simulink model "Crazyflie_TrajectoryTracking"  (R2020b)
settings: Solver=ode15s  StartTime=0.0  StopTime=100  MaxStep=1.0  RelTol=1e-5
settings Model: Creator=iketa  LastModifiedBy=kt012
settings DataIOCC: ReturnWorkspaceOutputs=off
settings DebuggingCC: ArithmeticOperatorsInVariantConditions=warning
settings SFSimCC: CustomCodeUndefinedFunction=UseInterfaceOnly

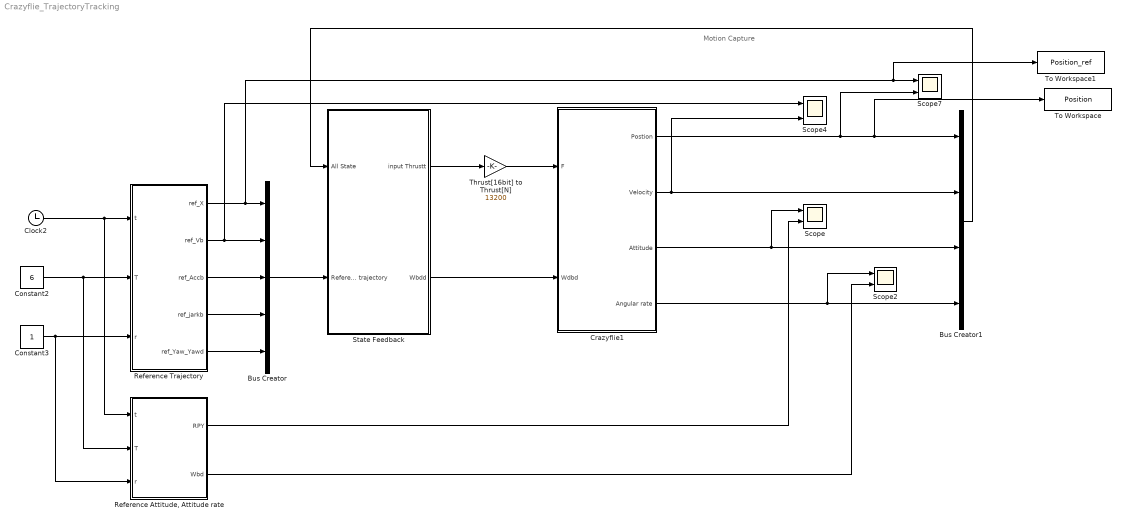
== system Crazyflie_TrajectoryTracking ==
  note: Motion Capture
  Bus Creator : BusCreator  Inputs=5
  Bus Creator1 : BusCreator  Inputs=Position,Body velosity,Euler_angle,Body anglar velosity
  Clock2 : Clock
  Constant2 : Constant  Value=6
  Constant3 : Constant
  Crazyflie1 : Subsystem
  "Reference Attitude, Attitude rate " : MATLAB Function  TreatAsAtomicUnit=on
  Reference Trajectory : MATLAB Function  TreatAsAtomicUnit=on
  Scope{,2,4,7} (4 alike) : Scope  NumInputPorts=2
  State Feedback : Subsystem
  Thrust[16bit] to Thrust[N] : Gain  Gain=13200
  To Workspace : ToWorkspace  VariableName=Position  SaveFormat=Timeseries  SampleTime=-1
  To Workspace1 : ToWorkspace  VariableName=Position_ref  SaveFormat=Timeseries  SampleTime=-1
  wires:
  Crazyflie1/2(Velocity) -> Bus Creator1/2, Scope4/2
  State Feedback/2("Wbdd ") -> Crazyflie1/2(Wdbd)
  Crazyflie1/3(Attitude) -> Scope/1, Bus Creator1/3
  Crazyflie1/4(Angular rate) -> Bus Creator1/4, Scope2/1
  Crazyflie1/1(Postion) -> Scope7/2, Bus Creator1/1, To Workspace/1
  Constant2/1 -> Reference Trajectory/2(T), "Reference Attitude, Attitude rate "/2(T)
  Constant3/1 -> Reference Trajectory/3(r), "Reference Attitude, Attitude rate "/3(r)
  Clock2/1 -> Reference Trajectory/1(t), "Reference Attitude, Attitude rate "/1(t)
  Reference Trajectory/3(ref_Accb) -> Bus Creator/3
  Bus Creator1/1 -> State Feedback/1(All State)
  Reference Trajectory/2(ref_Vb) -> Scope4/1, Bus Creator/2
  Reference Trajectory/1(ref_X) -> To Workspace1/1, Scope7/1, Bus Creator/1
  Thrust[16bit] to Thrust[N]/1 -> Crazyflie1/1(F)
  Reference Trajectory/5(ref_Yaw_Yawd) -> Bus Creator/5
  Bus Creator/1 -> State Feedback/2(Reference trajectory)
  State Feedback/1(input Thrustt) -> Thrust[16bit] to Thrust[N]/1
  Reference Trajectory/4(ref_jarkb) -> Bus Creator/4
  "Reference Attitude, Attitude rate "/2(Wbd) -> Scope2/2
  "Reference Attitude, Attitude rate "/1(RPY) -> Scope/2

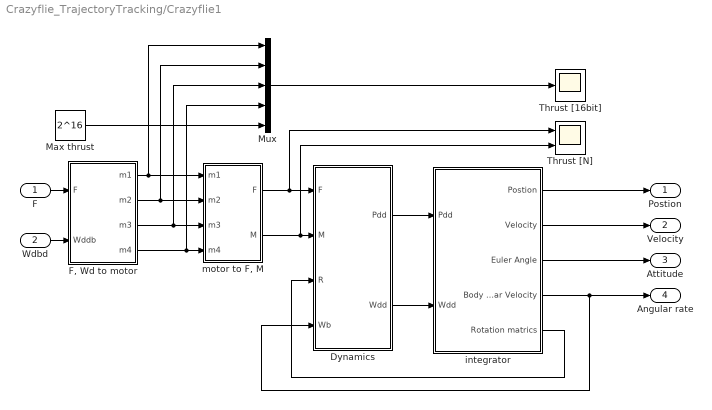
== system Crazyflie_TrajectoryTracking/Crazyflie1 ==
  F : Inport
  Wdbd : Inport  Port=2
  Dynamics : MATLAB Function  TreatAsAtomicUnit=on
  "F, Wd to motor" : MATLAB Function  TreatAsAtomicUnit=on
  Max thrust : Constant  Value=2^16
  Mux : Mux  Inputs=5
  "Thrust [16bit] " : Scope
  Thrust [N] : Scope  NumInputPorts=2
  integrator : Subsystem
  "motor to F, M" : MATLAB Function  TreatAsAtomicUnit=on
  Postion : Outport
  Velocity : Outport  Port=2
  Attitude : Outport  Port=3
  Angular rate : Outport  Port=4
  wires:
  "F, Wd to motor"/1(m1) -> "motor to F, M"/1(m1), Mux/1
  Wdbd/1 -> "F, Wd to motor"/2(Wddb)
  "F, Wd to motor"/4(m4) -> Mux/4, "motor to F, M"/4(m4)
  "F, Wd to motor"/2(m2) -> "motor to F, M"/2(m2), Mux/2
  "F, Wd to motor"/3(m3) -> "motor to F, M"/3(m3), Mux/3
  Dynamics/2(Wdd) -> integrator/2(Wdd)
  "motor to F, M"/2(M) -> Thrust [N]/2, Dynamics/2(M)
  integrator/4(Body Angular Velocity) -> Dynamics/4(Wb), Angular rate/1
  "motor to F, M"/1(F) -> Thrust [N]/1, Dynamics/1(F)
  F/1 -> "F, Wd to motor"/1(F)
  Dynamics/1(Pdd) -> integrator/1(Pdd)
  integrator/1(Postion) -> Postion/1
  integrator/2(Velocity) -> Velocity/1
  Mux/1 -> "Thrust [16bit] "/1
  Max thrust/1 -> Mux/5
  integrator/5(Rotation matrics) -> Dynamics/3(R)
  integrator/3(Euler Angle) -> Attitude/1

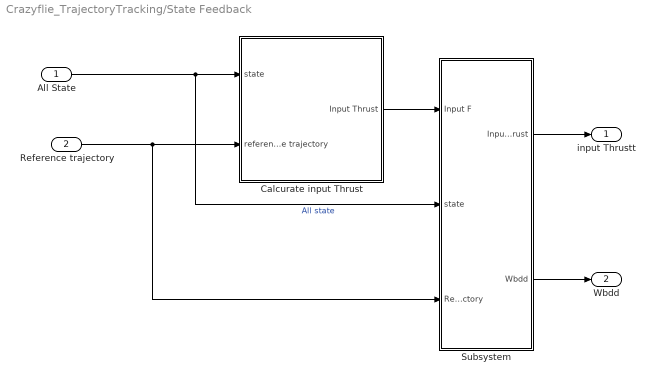
== system Crazyflie_TrajectoryTracking/State Feedback ==
  All State : Inport
  Reference trajectory : Inport  Port=2
  Calcurate input Thrust : Subsystem
  Subsystem : Subsystem
  input Thrustt : Outport
  "Wbdd " : Outport  Port=2  VectorParamsAs1DForOutWhenUnconnected=off
  wires:
  All State/1 -> Subsystem/2(state), Calcurate input Thrust/1(state)  "All state"
  Reference trajectory/1 -> Subsystem/3(Reference Trajectory), Calcurate input Thrust/2(reference trajectory)
  Calcurate input Thrust/1(Input Thrust) -> Subsystem/1(Input F)
  Subsystem/2("Wbdd ") -> "Wbdd "/1
  Subsystem/1(Input Thrust) -> input Thrustt/1

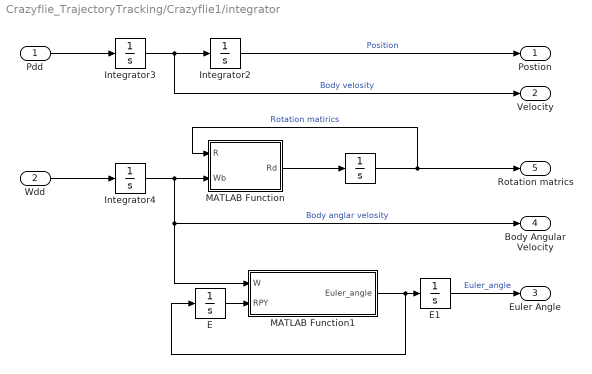
== system Crazyflie_TrajectoryTracking/Crazyflie1/integrator ==
  Pdd : Inport
  Wdd : Inport  Port=2
  " " : Integrator  InitialCondition=[1 0 0; 0 1 0; 0 0 1];  ContinuousStateAttributes="\"\""
  E : Integrator  InitialCondition=[0 0 0];
  E1 : Integrator  InitialCondition=[0 0 0];
  Integrator2 : Integrator  InitialCondition=[0 0.5 0];
  Integrator3 : Integrator  InitialCondition=[0 0 0.0];
  Integrator4 : Integrator  InitialCondition=[0 0 0];  ContinuousStateAttributes='Body_anglar_velocity'
  MATLAB Function : MATLAB Function  TreatAsAtomicUnit=on
  MATLAB Function1 : MATLAB Function  TreatAsAtomicUnit=on
  Postion : Outport
  Velocity : Outport  Port=2
  Euler Angle : Outport  Port=3
  Body Angular Velocity : Outport  Port=4
  Rotation matrics : Outport  Port=5
  wires:
  Integrator4/1 -> Body Angular Velocity/1, MATLAB Function1/1(W), MATLAB Function/2(Wb)  "Body anglar velosity"
  Pdd/1 -> Integrator3/1
  Integrator3/1 -> Integrator2/1, Velocity/1  "Body velosity"
  Integrator2/1 -> Postion/1  "Position"
  Wdd/1 -> Integrator4/1
  " "/1 -> MATLAB Function/1(R), Rotation matrics/1  "Rotation matirics"
  MATLAB Function/1(Rd) -> " "/1
  E/1 -> MATLAB Function1/2(RPY)
  MATLAB Function1/1(Euler_angle) -> E/1, E1/1
  E1/1 -> Euler Angle/1  "Euler_angle"

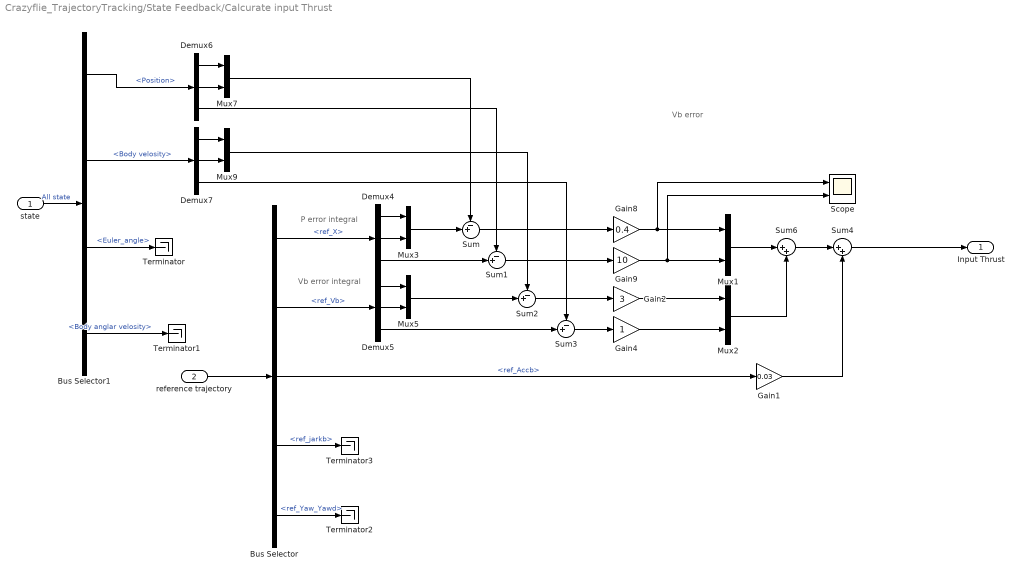
== system Crazyflie_TrajectoryTracking/State Feedback/Calcurate input Thrust ==
  note: Vb error
  note: P error integral
  note: Vb error integral
  state : Inport
  reference trajectory : Inport  Port=2
  Bus Selector : BusSelector  OutputSignals=ref_X,ref_Vb,ref_Accb,ref_jarkb,ref_Yaw_Yawd
  Bus Selector1 : BusSelector  OutputSignals=Position,Body velosity,Euler_angle,Body anglar velosity
  Demux{4..7} (4 alike) : Demux  Outputs=3
  Gain1 : Gain  Gain=0.03
  Gain2 : Gain  Gain=3
  Gain4 : Gain
  Gain8 : Gain  Gain=0.4
  Gain9 : Gain  Gain=10
  Mux{1..3,5,7,9} (6 alike) : Mux  Inputs=2
  Scope : Scope  NumInputPorts=2
  Sum{,1..3} (4 alike) : Sum  Inputs=-+|
  Sum4 : Sum  Inputs=|++
  Sum6 : Sum  Inputs=|++
  Terminator{,1..3} (4 alike) : Terminator
  Input Thrust : Outport
  wires:
  Gain9/1 -> Scope/2, Mux1/2
  Demux5/1 -> Mux5/1
  Gain8/1 -> Scope/1, Mux1/1
  Demux7/3 -> Sum3/1
  Bus Selector/2 -> Demux5/1  "<ref_Vb>"
  Demux5/2 -> Mux5/2
  Mux7/1 -> Sum/1
  Mux9/1 -> Sum2/1
  Sum2/1 -> Gain2/1
  Sum6/1 -> Sum4/1
  Demux7/2 -> Mux9/2
  Demux4/2 -> Mux3/2
  Sum1/1 -> Gain9/1
  Demux6/2 -> Mux7/2
  Demux6/3 -> Sum1/1
  Gain4/1 -> Mux2/2
  Sum/1 -> Gain8/1
  Demux4/1 -> Mux3/1
  Mux2/1 -> Sum6/2
  Demux4/3 -> Sum1/2
  reference trajectory/1 -> Bus Selector/1
  Sum3/1 -> Gain4/1
  Gain2/1 -> Mux2/1
  Mux1/1 -> Sum6/1
  Demux6/1 -> Mux7/1
  Gain1/1 -> Sum4/2
  state/1 -> Bus Selector1/1  "All state"
  Bus Selector1/4 -> Terminator1/1  "<Body anglar velosity>"
  Bus Selector1/2 -> Demux7/1  "<Body velosity>"
  Mux5/1 -> Sum2/2
  Mux3/1 -> Sum/2
  Demux5/3 -> Sum3/2
  Bus Selector1/3 -> Terminator/1  "<Euler_angle>"
  Demux7/1 -> Mux9/1
  Bus Selector1/1 -> Demux6/1  "<Position>"
  Sum4/1 -> Input Thrust/1
  Bus Selector/3 -> Gain1/1  "<ref_Accb>"
  Bus Selector/1 -> Demux4/1  "<ref_X>"
  Bus Selector/5 -> Terminator2/1  "<ref_Yaw_Yawd>"
  Bus Selector/4 -> Terminator3/1  "<ref_jarkb>"

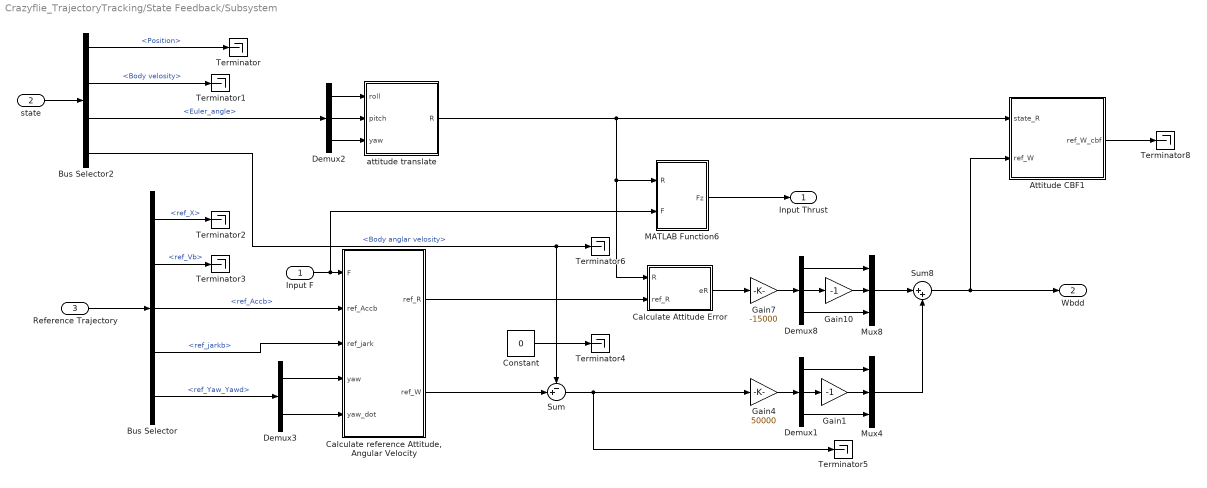
== system Crazyflie_TrajectoryTracking/State Feedback/Subsystem ==
  Input F : Inport
  state : Inport  Port=2
  Reference Trajectory : Inport  Port=3
  Attitude CBF1 : MATLAB Function  TreatAsAtomicUnit=on
  Bus Selector : BusSelector  OutputSignals=ref_X,ref_Vb,ref_Accb,ref_jarkb,ref_Yaw_Yawd
  Bus Selector2 : BusSelector  OutputSignals=Position,Body velosity,Euler_angle,Body anglar velosity
  Calculate Attitude Error : MATLAB Function  TreatAsAtomicUnit=on
  "Calculate reference Attitude, Angular Velocity" : MATLAB Function  TreatAsAtomicUnit=on
  Constant : Constant  Value=0
  Demux1 : Demux  Outputs=3
  Demux2 : Demux  Outputs=3
  Demux3 : Demux  Outputs=2
  Demux8 : Demux  Outputs=3
  Gain1 : Gain  Gain=-1
  Gain10 : Gain  Gain=-1
  Gain4 : Gain  Gain=50000
  Gain7 : Gain  Gain=-15000
  MATLAB Function6 : MATLAB Function
  Mux4 : Mux  Inputs=3
  Mux8 : Mux  Inputs=3
  Sum : Sum  Inputs=-+|
  Sum8 : Sum  Inputs=|++
  Terminator{,1..6,8} (8 alike) : Terminator
  attitude translate : MATLAB Function  TreatAsAtomicUnit=on
  Input Thrust : Outport
  "Wbdd " : Outport  Port=2  VectorParamsAs1DForOutWhenUnconnected=off
  wires:
  Sum/1 -> Gain4/1, Terminator5/1
  Mux4/1 -> Sum8/2
  Bus Selector/2 -> Terminator3/1  "<ref_Vb>"
  Demux8/3 -> Mux8/3
  "Calculate reference Attitude, Angular Velocity"/1(ref_R) -> Calculate Attitude Error/2(ref_R)
  Mux8/1 -> Sum8/1
  Sum8/1 -> "Wbdd "/1, Attitude CBF1/2(ref_W)
  Input F/1 -> MATLAB Function6/2(F), "Calculate reference Attitude, Angular Velocity"/1(F)
  Demux8/2 -> Gain10/1
  attitude translate/1(R) -> Attitude CBF1/1(state_R), Calculate Attitude Error/1(R), MATLAB Function6/1(R)
  Demux8/1 -> Mux8/1
  Gain10/1 -> Mux8/2
  Demux1/2 -> Gain1/1
  Bus Selector2/3 -> Demux2/1  "<Euler_angle>"
  Bus Selector2/2 -> Terminator1/1  "<Body velosity>"
  Bus Selector2/1 -> Terminator/1  "<Position>"
  Bus Selector/5 -> Demux3/1  "<ref_Yaw_Yawd>"
  Bus Selector2/4 -> Terminator6/1, Sum/1  "<Body anglar velosity>"
  Reference Trajectory/1 -> Bus Selector/1
  Bus Selector/3 -> "Calculate reference Attitude, Angular Velocity"/2(ref_Accb)  "<ref_Accb>"
  "Calculate reference Attitude, Angular Velocity"/2(ref_W) -> Sum/2
  Demux3/1 -> "Calculate reference Attitude, Angular Velocity"/4(yaw)
  Calculate Attitude Error/1(eR) -> Gain7/1
  Demux3/2 -> "Calculate reference Attitude, Angular Velocity"/5(yaw_dot)
  state/1 -> Bus Selector2/1
  MATLAB Function6/1(Fz) -> Input Thrust/1
  Bus Selector/1 -> Terminator2/1  "<ref_X>"
  Bus Selector/4 -> "Calculate reference Attitude, Angular Velocity"/3(ref_jark)  "<ref_jarkb>"
  Demux2/1 -> attitude translate/1(roll)
  Demux2/2 -> attitude translate/2(pitch)
  Demux2/3 -> attitude translate/3(yaw)
  Gain7/1 -> Demux8/1
  Demux1/1 -> Mux4/1
  Demux1/3 -> Mux4/3
  Gain4/1 -> Demux1/1
  Gain1/1 -> Mux4/2
  Constant/1 -> Terminator4/1
  Attitude CBF1/1(ref_W_cbf) -> Terminator8/1

== matlab function Crazyflie_TrajectoryTracking/Crazyflie1/motor to F, M ==
  data: F output; m1 input; m2 input; M output; m3 input; m4 input
function [F, M] = func(m1, m2, m3, m4)

% F [16bit] Wddb [16bit]

Armlength = 0.035;
m1 = 2.130295 * 10^(-11) * m1^2 + 1.032633 * 10^(-6) * m1 + 5.484560 * 10^(-4);
m2 = 2.130295 * 10^(-11) * m2^2 + 1.032633 * 10^(-6) * m2 + 5.484560 * 10^(-4);
m3 = 2.130295 * 10^(-11) * m3^2 + 1.032633 * 10^(-6) * m3 + 5.484560 * 10^(-4);
m4 = 2.130295 * 10^(-11) * m4^2 + 1.032633 * 10^(-6) * m4 + 5.484560 * 10^(-4);

% calculate thrust
F = m1 + m2 + m3 + m4;

% calculate moment formation X
M1 = Armlength / sqrt(2) * (m3 + m4 - m1 - m2);
M2 = -Armlength / sqrt(2) * (-m3 - m2 + m1 + m4);

% calculate moment formation + 
% M1 = Armlength  * (m4 - m2);
% M2 = Armlength * (m1 - m3);

M3 = m1 + m3 - m2 - m4;

M = [M1 M2 M3]';

== matlab function Crazyflie_TrajectoryTracking/Crazyflie1/integrator/MATLAB Function ==
  data: R input; Rd output; Wb input
function Rd = fcn(R, Wb)
wx = Wb(1);
wy = Wb(2);
wz = Wb(3);
Wb = [ 0    -wz   wy;
       wz    0   -wx;
      -wy    wx   0];
Rd = R * Wb;

== matlab function Crazyflie_TrajectoryTracking/Reference Trajectory ==
  data: ref_X output; ref_Vb output; ref_Accb output; ref_jarkb output; t input; T input; r input; ref_Yaw_Yawd output
function [ref_X, ref_Vb, ref_Accb, ref_jarkb, ref_Yaw_Yawd] = fcn(t,T,r)
% 軌道生成
w = 2 * pi/T;          % 角周波数

% 中心　半径　　
c = [0;0;0];

ref_X = c + r*[sin(w*t); cos(w*t); 0];
ref_Vb = r*[w*cos(w*t); -w*sin(w*t); 0];
ref_Accb = [-r*w^2*sin(w*t); -r*w^2*cos(w*t); 9.8];
ref_jarkb = r*[-w^3*cos(w*t); w^3*sin(w*t); 0];
ref_Yaw_Yawd = [0, 0]';

== matlab function Crazyflie_TrajectoryTracking/State Feedback/Subsystem/attitude translate ==
  data: roll input; R output; pitch input; yaw input
function R = fcn(roll, pitch, yaw)
% RPYから回転行列計算

R3 = [ cos(yaw) -sin(yaw) 0; sin(yaw) cos(yaw) 0; 0 0 1];              % ヨー角
R2 = [ cos(pitch) 0 sin(pitch); 0 1 0; -sin(pitch) 0 cos(pitch) ];     % ピッチ角
R1 = [ 1 0 0; 0 cos(roll) -sin(roll); 0 sin(roll) cos(roll)];          % ロール角

R = R3* R2 * R1;   % 回転行列（ボディー　-> ワールド）3

== matlab function Crazyflie_TrajectoryTracking/State Feedback/Subsystem/Calculate reference Attitude, Angular Velocity ==
  data: ref_R output; ref_W output; F input; ref_Accb input; ref_jark input; yaw input; yaw_dot input
function [ref_R, ref_W]= fcn(F, ref_Accb, ref_jark, yaw, yaw_dot)

% Flat Outputから内部状態と入力揚力を計算

m = 0.03;
F = F;
Xc = [cos(yaw) sin(yaw) 0]';          % よー角のベクトル　Rc(3)
Yc = [-sin(yaw) cos(yaw) 0]';
dXc = yaw_dot * Yc; % よー角のベクトルの微分
dYc = -yaw_dot * Xc; 

% 所望の姿勢を計算している
% 軌道の加速度のベクトル: b3 を計算
Zb = F / norm(F);   
%
Xb = cross(Yc, Zb)/norm(cross(Yc, Zb));
Yb = cross(Zb, Xb);
ref_R = [Xb Yb Zb] ;

% 加加速度ベクトルを計算
dfZb = ref_jark;
  
% 目標の姿勢のz軸方向のベクトルの微分を計算
dZb = dfZb/norm(F) - F * dot(F, dfZb)/norm(F)^3; % Zb_dot---------- dot(　fb1/norm(fb1) )

% 目標の姿勢のx軸方向のベクトルを計算
dnorm_Zb_Xc2 = norm(cross(dYc, Zb) + cross(Yc, dZb));
dXb = (cross(dYc, Zb) + cross(Yc, dZb))/dnorm_Zb_Xc2 - cross(Yc, Zb) * dot(cross(Yc, Zb),( cross(dYc, Zb) + cross(Yc, dZb)))/dnorm_Zb_Xc2^3;
   
% 目標の姿勢のy軸方向のベクトルを計算
dYb = cross(dZb, Xb) + cross(Zb, dXb) ;  %dot_b2 = dotb3とb1 の外積と　b3とdot_b1の外積　の和　--------- dot(cross(b3, b1))


wy = dot(Xb, ref_jark) / dot(Zb, ref_Accb);
wx = - dot(Yb, ref_jark) / dot(Zb, ref_Accb);
wz = (yaw_dot * dot(Xc, Xb) + wy * dot(Yb, Zb))/norm(cross(Yc, Zb));
ref_W = [wx wy wz];

== matlab function Crazyflie_TrajectoryTracking/State Feedback/Subsystem/Calculate Attitude Error ==
  data: R input; ref_R input; eR output
function eR = fcn(R, ref_R)
transpose_R = R';
transpose_ref_R = ref_R';
tmp = (transpose_ref_R*R - transpose_R*ref_R)/2;
eR = [tmp(3, 2), -tmp(3, 1), tmp(2, 1)];

== matlab function Crazyflie_TrajectoryTracking/State Feedback/Subsystem/MATLAB Function6 ==
  data: R input; F input; Fz output
function Fz = fcn(R, F)
e3 = [0;0;1];
u = dot(F, R*e3);

Fz = u;

== matlab function Crazyflie_TrajectoryTracking/Reference Attitude, Attitude rate  ==
  data: RPY output; Wbd output; t input; T input; r input
function [RPY, Wbd] = fcn(t,T,r)
% 軌道生成
w = 2 * pi/T;          % 角周波数

% 中心　半径　　
c = [0;0;0];

% Flat Outputから内部状態と入力揚力を計算
% 各軸の単位行列
e1 = [1; 0; 0];e2 = [0; 1; 0];e3 = [0; 0; 1];
% ドローンの質量　重力加速度
mQ = 0.027; g = 9.8;


x = c + r*[sin(w*t); cos(w*t); 0];         % 位置の軌道の位置
dx = r*[w*cos(w*t); -w*sin(w*t); 0];       % 速度の軌道
d2x = r*[-w^2*sin(w*t); -w^2*cos(w*t); 0]; % 加速度の軌道
d3x = r*[-w^3*cos(w*t); w^3*sin(w*t); 0];  % 加加速度の軌道
d4x = r*[w^4*sin(w*t); w^4*cos(w*t); 0];   % 加加加速度の軌道

alpha = 0;                                 
d_alpha = 0;                               
d2x(3) = d2x(3)+g;

pitch = atan( ( d2x(1)*cos(alpha) + d2x(2)*sin(alpha) ) / (d2x(3)));                                                        
roll = atan( ( d2x(1)*sin(alpha) - d2x(2)*cos(alpha) ) / sqrt( (d2x(3))^2 + ( d2x(1)*cos(alpha) + d2x(2)*sin(alpha) )^2));

rollS = sin(roll); rollC = cos(roll);           
pitchS = sin(pitch); pitchC = cos(pitch);       
yawS = sin(alpha); yawC = cos(alpha);           


% desired Roll rate
roll_rate_bunshi = d2x(3)^2 * ( d3x(1)*yawS - d3x(2)*yawC + d_alpha * (d2x(1)*yawC + d2x(2)*yawS) ) - d2x(3)*d3x(3)*(d2x(1)*yawS - d2x(2)*yawC) + (d2x(1)*yawC + d2x(2)*yawS)*(d_alpha*(d2x(1)^2 + d2x(2)^2) - d2x(1)*d3x(2) + d2x(2)*d3x(1));
roll_rate_bunbo = (d2x(1)^2 + d2x(2)^2 + d2x(3)^2) * sqrt(d2x(3)^2 + ( d2x(1)*yawC + d2x(2)*yawS )^2);
roll_rate = roll_rate_bunshi / roll_rate_bunbo;

% desired Pitch rate
pitch_rate_bunshi = d2x(3)*(d3x(1)*yawC + d3x(2)*yawS) - d3x(3)*(d2x(1)*yawC + d2x(2)*yawS) - d2x(3)*d_alpha*(d2x(1)*yawS + d2x(2)*yawC);
pitch_rate_bunbo = d2x(3)^2 + ( d2x(1)*yawC + d2x(2)*yawS )^2;
pitch_rate = pitch_rate_bunshi / pitch_rate_bunbo;

W = [1 0      -pitchS;
     0 rollC  pitchC * rollS;
     0 -rollS pitchC * rollC] * [roll_rate;pitch_rate;d_alpha];

RPY = [roll, pitch, alpha]';
Wbd = W;

== matlab function Crazyflie_TrajectoryTracking/State Feedback/Subsystem/Attitude CBF1 ==
  data: state_R input; ref_W input; ref_W_cbf output
function ref_W_cbf = fcn(state_R, ref_W)
theta = 0.2;
coder.extrinsic('quadprog')
tmp = zeros(3, 1);
e3 = [0; 0; 1];
e3_wedge = [0 -1 0; 1 0 0; 0 0 0];
H = eye(3);
f = -2*ref_W;
% ref_W
A = e3'*state_R*e3_wedge;
B = (e3'*state_R*e3 - cos(theta));



tmp  = quadprog(H, f, A, B);
ref_W_cbf = [0      -tmp(3)   tmp(2); 
             tmp(3)  0       -tmp(1); 
             -tmp(2) tmp(1)   0];
if A * tmp > B
    A * tmp
    B
end

== matlab function Crazyflie_TrajectoryTracking/Crazyflie1/Dynamics ==
  data: Pdd output; F input; M input; R input; Wb input; Wdd output
function [Pdd,Wdd] = fcn(F, M, R, Wb)
m = 0.03;
e3 = [0 0 1]';
g = 9.8;
% % crazyflie
I = [16.571710 0.830806 0.718277;
     0.830806 16.655602 1.800197;
     0.718277 1.800197 29.261652] * 10^(-6);      % crazyflieの慣性モーメント（kg・m^2）
I = [1 0 0;
     0 1 0;
     0 0 1] * 10^(-6);
% 機体上向き加速度
Pdd = (F * R*e3 - m*g*e3)/m;

% 各加速度計算（ボディー座標系）
Wdd = pinv(I)*(M - cross(Wb, I * Wb));

== matlab function Crazyflie_TrajectoryTracking/Crazyflie1/F, Wd to motor ==
  data: F input; Wddb input; m1 output; m2 output; m3 output; m4 output
 function [m1, m2, m3, m4]= fcn(F, Wddb)

% F [16bit] Wddb [16bit]

r = min(max(-32000, Wddb(1)), 32000)/2;
p = min(max(-32000, Wddb(2)), 32000)/2;
y = min(max(-32000, Wddb(3)), 32000);

m1 = min(max(0,F - r + p + y), 2^16);
m2 = min(max(0,F - r - p - y), 2^16);
m3 = min(max(0,F + r - p + y), 2^16);
m4 = min(max(0,F + r + p - y), 2^16);

% formation +
% r = min(max(-32000, Wddb(1)), 32000);
% p = min(max(-32000, Wddb(2)), 32000);
% y = min(max(-32000, Wddb(3)), 32000);
% m1 = min(max(0, + p + y), 2^16);
% m2 = min(max(0, - r - y), 2^16);
% m3 = min(max(0, - p + y), 2^16);
% m4 = min(max(0, + r - y), 2^16);

%         ^y
%         |
%         |
%   m3          m4
%
%                    ------>x
%
%   m2          m1

== matlab function Crazyflie_TrajectoryTracking/Crazyflie1/integrator/MATLAB Function1 ==
  data: W input; Euler_angle output; RPY input
function Euler_angle = fcn(W, RPY)
roll = RPY(1);
pitch = RPY(2);
yaw = RPY(3);
rollS = sin(roll); rollC = cos(roll);           
pitchS = sin(pitch); pitchC = cos(pitch);       


Euler_angle = pinv([1 0 -pitchS;
     0 rollC  pitchC * rollS;
     0 -rollS pitchC * rollC]) * W;
